simulink model "INTERLOCK_DELAY_Flex2"  (R2016a)
settings: Solver=FixedStepDiscrete  StartTime=0.0  StopTime=10.0  RelTol=1e-3
values from neighbouring files (symbols this model uses):
  DELAY_COUNT = 25    [Init_InterLock.m]
  INVERSE_BOTTOMSWITCH = 0    [Init_InterLock.m]
undefined symbols (not defined in the file or in its folder): DelayCount, sigbuilder_block
libraries: simulink x6
settings Model: Creator=zedboard  LastModifiedBy=Wendel
settings OptimizationCC: BlockReduction=off  ConditionallyExecuteInputs=off  DefaultParameterBehavior=Inlined
settings DebuggingCC: AlgebraicLoopMsg=error
settings HardwareCC: ProdBitPerPointer=32  ProdLargestAtomicFloat=None  ProdIntDivRoundTo=Undefined  ProdEndianess=Unspecified  ProdWordSize=32  ProdHWDeviceType=ASIC/FPGA->ASIC/FPGA  ProdEqTarget=off

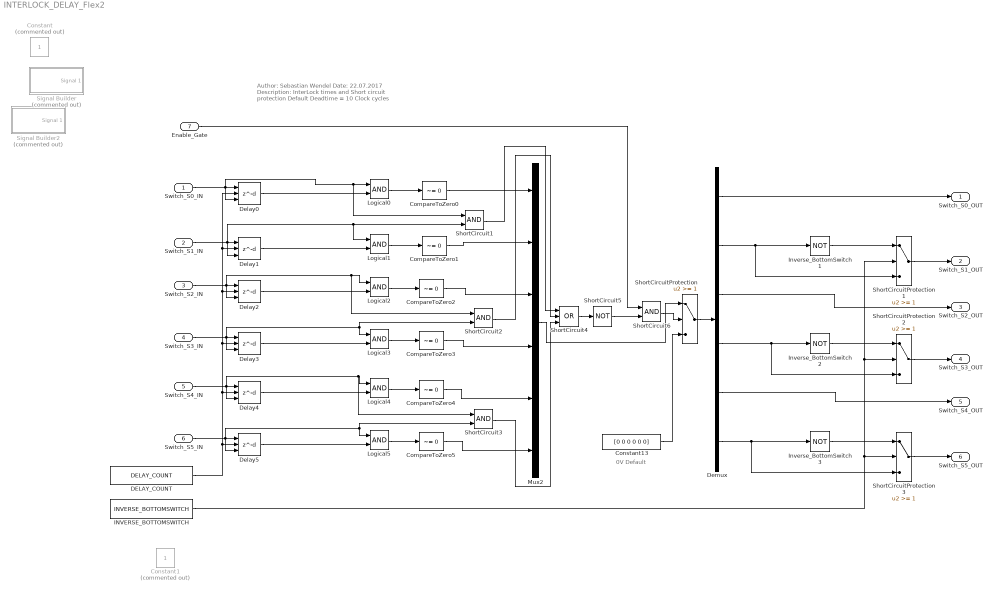
== system INTERLOCK_DELAY_Flex2 ==
  note: Author: Sebastian Wendel
      | Date: 22.07.2017
      | Description:
      | InterLock times and Short circuit protection
      | Default Deadtime = 10 Clock cycles
  note: 0V Default
  Switch_S0_IN : Inport  OutDataTypeStr=boolean
  Switch_S1_IN : Inport  Port=2  OutDataTypeStr=boolean
  Switch_S2_IN : Inport  Port=3  OutDataTypeStr=boolean
  Switch_S3_IN : Inport  Port=4  OutDataTypeStr=boolean
  Switch_S4_IN : Inport  Port=5  OutDataTypeStr=boolean
  Switch_S5_IN : Inport  Port=6  OutDataTypeStr=boolean
  Enable_Gate : Inport  Port=7  OutDataTypeStr=boolean
  CompareToZero{0..5} (6 alike) : simulink/Logic and Bit Operations/Compare To Zero  relop=~=  OutDataTypeStr=boolean
  Constant : Constant  Commented=on
  Constant1 : Constant  Commented=on
  Constant13 : Constant  Value=[0 0 0 0 0 0]  OutDataTypeStr=boolean  SampleTime=-1
  DELAY_COUNT : Constant  Value=DELAY_COUNT  OutDataTypeStr=int8  SampleTime=-1
  Delay0 : Delay  DelayLengthSource=Input port  DelayLength=DelayCount  InitialCondition=0  ExternalReset=Falling  RemoveProtectionDelayLength=on
      settings: InputPortMap=u0,p1,r5
  Delay1 : Delay  DelayLengthSource=Input port  DelayLength=DelayCount  InitialCondition=0  ExternalReset=Falling  InputProcessing=Columns as channels (frame based)
      settings: InputPortMap=u0,p1,r5
  Delay2 : Delay  DelayLengthSource=Input port  DelayLength=DelayCount  InitialCondition=0  ExternalReset=Falling  InputProcessing=Inherited
      settings: InputPortMap=u0,p1,r5
  Delay3 : Delay  DelayLengthSource=Input port  DelayLength=DelayCount  InitialCondition=0  ExternalReset=Falling
      settings: InputPortMap=u0,p1,r5
  Delay4 : Delay  DelayLengthSource=Input port  DelayLength=DelayCount  InitialCondition=0  ExternalReset=Falling
      settings: InputPortMap=u0,p1,r5
  Delay5 : Delay  DelayLengthSource=Input port  DelayLength=DelayCount  InitialCondition=0  ExternalReset=Falling
      settings: InputPortMap=u0,p1,r5
  Demux : Demux  Outputs=6
  INVERSE_BOTTOMSWITCH : Constant  Value=INVERSE_BOTTOMSWITCH  OutDataTypeStr=boolean  SampleTime=-1
  Inverse_BottomSwitch1 : Logic  Operator=NOT  Inputs=3  AllPortsSameDT=off  OutDataTypeStr=boolean
  Inverse_BottomSwitch2 : Logic  Operator=NOT  Inputs=3  AllPortsSameDT=off  OutDataTypeStr=boolean
  Inverse_BottomSwitch3 : Logic  Operator=NOT  Inputs=3  AllPortsSameDT=off  OutDataTypeStr=boolean
  Logical{0..5} (6 alike) : Logic  AllPortsSameDT=off  OutDataTypeStr=boolean
  Mux2 : Mux  Inputs=6
  ShortCircuit{1..3,6} (4 alike) : Logic  AllPortsSameDT=off  OutDataTypeStr=boolean
  ShortCircuit4 : Logic  Operator=OR  Inputs=3  AllPortsSameDT=off  OutDataTypeStr=boolean
  ShortCircuit5 : Logic  Operator=NOT  Inputs=3  AllPortsSameDT=off  OutDataTypeStr=boolean
  ShortCircuitProtection{,1..3} (4 alike) : Switch  Threshold=1
  Signal Builder : Subsystem  Tag=STV Subsys  Commented=on  LoadFcn=sigbuilder_block('load');  StartFcn=sigbuilder_block('start');  StopFcn=sigbuilder_block('stop');  ClipboardFcn=sigbuilder_block('clipboard');  mask(Sigbuilder block){}
      mask help: Simulink:masks:SigbuilderBlock_MD
      mask init:
      | if ~strcmp(get_param(bdroot(gcbh),'SimulationStatus'),'stopped') tuvar = sigbuilder_block('maskInit'); end
      settings: CopyFcn=sigbuilder_block('copy');  DeleteFcn=sigbuilder_block('delete');  ModelCloseFcn=sigbuilder_block('modelClose');  PreSaveFcn=sigbuilder_block('preSave');  PauseFcn=sigbuilder_block('pause');  ContinueFcn=sigbuilder_block('continue');  NameChangeFcn=sigbuilder_block('namechange');  OpenFcn=sigbuilder_block('open',[595.8 39 550.8 361.2 ]);  CloseFcn=sigbuilder_block('close');
      mask Display: plot(0, 0, 100, 100,[2, 2, 32, 32, 2], [68, 8, 8, 68, 68],[32, 2], [38, 38], [32, 19, 2],[53, 60, 44], [32, 17, 17, 2],[16, 16, 31, 31]);txt = getActiveGroup(gcbh);text(2, 100, txt,'verticalAlignment', 'top');
  Signal Builder2 : Subsystem  Tag=STV Subsys  Commented=on  LoadFcn=sigbuilder_block('load');  StartFcn=sigbuilder_block('start');  StopFcn=sigbuilder_block('stop');  ClipboardFcn=sigbuilder_block('clipboard');  mask(Sigbuilder block){}
      mask help: Simulink:masks:SigbuilderBlock_MD
      mask init:
      | if ~strcmp(get_param(bdroot(gcbh),'SimulationStatus'),'stopped') tuvar = sigbuilder_block('maskInit'); end
      settings: CopyFcn=sigbuilder_block('copy');  DeleteFcn=sigbuilder_block('delete');  ModelCloseFcn=sigbuilder_block('modelClose');  PreSaveFcn=sigbuilder_block('preSave');  PauseFcn=sigbuilder_block('pause');  ContinueFcn=sigbuilder_block('continue');  NameChangeFcn=sigbuilder_block('namechange');  OpenFcn=sigbuilder_block('open',[437.6 199.2 550.4 400 ]);  CloseFcn=sigbuilder_block('close');
      mask Display: plot(0, 0, 100, 100,[2, 2, 32, 32, 2], [68, 8, 8, 68, 68],[32, 2], [38, 38], [32, 19, 2],[53, 60, 44], [32, 17, 17, 2],[16, 16, 31, 31]);txt = getActiveGroup(gcbh);text(2, 100, txt,'verticalAlignment', 'top');
  Switch_S0_OUT : Outport
  Switch_S1_OUT : Outport  Port=2
  Switch_S2_OUT : Outport  Port=3
  Switch_S3_OUT : Outport  Port=4
  Switch_S4_OUT : Outport  Port=5
  Switch_S5_OUT : Outport  Port=6
  wires:
  Delay0/1 -> Logical0/2
  Logical0/1 -> CompareToZero0/1
  CompareToZero0/1 -> Mux2/1
  Enable_Gate/1 -> ShortCircuit6/1
  Delay1/1 -> Logical1/2
  Logical1/1 -> CompareToZero1/1
  CompareToZero1/1 -> Mux2/2
  Switch_S2_IN/1 -> Delay2/3, ShortCircuit2/1, Logical2/1, Delay2/1
  Delay2/1 -> Logical2/2
  Logical2/1 -> CompareToZero2/1
  CompareToZero2/1 -> Mux2/3
  Switch_S3_IN/1 -> Delay3/3, ShortCircuit2/2, Logical3/1, Delay3/1
  Delay3/1 -> Logical3/2
  Logical3/1 -> CompareToZero3/1
  CompareToZero3/1 -> Mux2/4
  Switch_S4_IN/1 -> Delay4/3, ShortCircuit3/1, Logical4/1, Delay4/1
  Delay4/1 -> Logical4/2
  Logical4/1 -> CompareToZero4/1
  CompareToZero4/1 -> Mux2/5
  Switch_S5_IN/1 -> Delay5/1, Delay5/3, ShortCircuit3/2, Logical5/1
  Delay5/1 -> Logical5/2
  Logical5/1 -> CompareToZero5/1
  CompareToZero5/1 -> Mux2/6
  Mux2/1 -> ShortCircuitProtection/1
  Constant13/1 -> ShortCircuitProtection/3
  ShortCircuitProtection/1 -> Demux/1
  Demux/2 -> ShortCircuitProtection1/3, Inverse_BottomSwitch1/1
  Demux/3 -> Switch_S2_OUT/1
  Demux/5 -> Switch_S4_OUT/1
  ShortCircuit4/1 -> ShortCircuit5/1
  ShortCircuit1/1 -> ShortCircuit4/1
  ShortCircuit2/1 -> ShortCircuit4/2
  ShortCircuit3/1 -> ShortCircuit4/3
  Switch_S1_IN/1 -> Logical1/1, ShortCircuit1/2, Delay1/3, Delay1/1
  ShortCircuit6/1 -> ShortCircuitProtection/2
  ShortCircuit5/1 -> ShortCircuit6/2
  Inverse_BottomSwitch1/1 -> ShortCircuitProtection1/1
  ShortCircuitProtection1/1 -> Switch_S1_OUT/1
  Demux/4 -> ShortCircuitProtection2/3, Inverse_BottomSwitch2/1
  Inverse_BottomSwitch2/1 -> ShortCircuitProtection2/1
  ShortCircuitProtection2/1 -> Switch_S3_OUT/1
  Demux/6 -> Inverse_BottomSwitch3/1, ShortCircuitProtection3/3
  Inverse_BottomSwitch3/1 -> ShortCircuitProtection3/1
  ShortCircuitProtection3/1 -> Switch_S5_OUT/1
  INVERSE_BOTTOMSWITCH/1 -> ShortCircuitProtection1/2, ShortCircuitProtection2/2, ShortCircuitProtection3/2
  Switch_S0_IN/1 -> Delay0/3, Delay0/1, ShortCircuit1/1, Logical0/1
  Demux/1 -> Switch_S0_OUT/1
  DELAY_COUNT/1 -> Delay0/2, Delay1/2, Delay2/2, Delay3/2, Delay4/2, Delay5/2

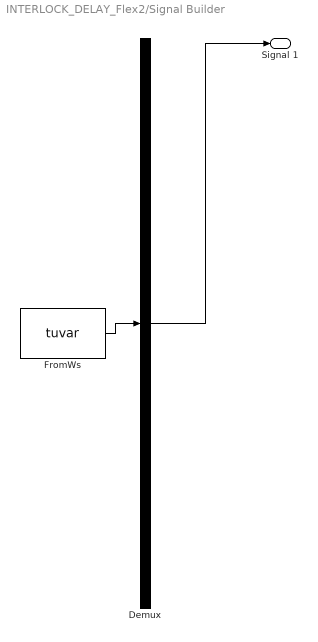
== system INTERLOCK_DELAY_Flex2/Signal Builder ==
  Demux : Demux  Tag=STV Demux  Outputs=1
  FromWs : FromWorkspace  Tag=STV FromWs  VariableName=tuvar  SampleTime=0
      SigBuilderData=|
      | common.afterFinalStr = 'Extrapolate'
      | common.sampleTime = 0
      | dataSet.timeRange = [0 10]
      | dataSet.name = 'Group 1'
      | sbobj.Groups.Name = 'Group 1'
      | sbobj.Groups.Signals.Name = 'Signal 1'
      | sbobj.Groups.Signals.XData = [0 1.02 1.02 6 6 10]
      | sbobj.Groups.Signals.YData = [0 0 1 1 0 0]
  Signal 1 : Outport  Tag=STV Outport
  wires:
  Demux/1 -> Signal 1/1
  FromWs/1 -> Demux/1

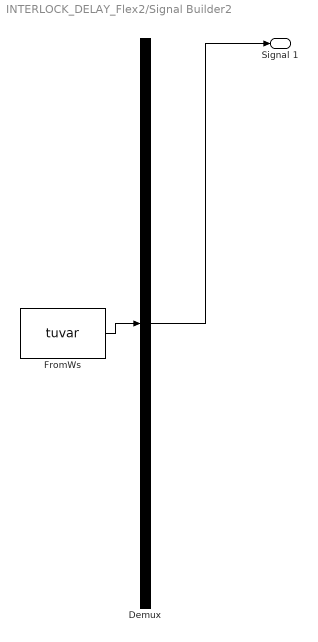
== system INTERLOCK_DELAY_Flex2/Signal Builder2 ==
  Demux : Demux  Tag=STV Demux  Outputs=1
  FromWs : FromWorkspace  Tag=STV FromWs  VariableName=tuvar  SampleTime=0
      SigBuilderData=|
      | common.afterFinalStr = 'Extrapolate'
      | common.sampleTime = 0
      | dataSet.timeRange = [0 10]
      | dataSet.name = 'Group 1'
      | sbobj.Groups.Name = 'Group 1'
      | sbobj.Groups.Signals.Name = 'Signal 1'
      | sbobj.Groups.Signals.XData = [0 1.9 1.9 8 8 10]
      | sbobj.Groups.Signals.YData = [0 0 1 1 0 0]
  Signal 1 : Outport  Tag=STV Outport
  wires:
  Demux/1 -> Signal 1/1
  FromWs/1 -> Demux/1
